simulink model "Swarm"  (Simulink 7.7)
settings: Solver=ode5  StartTime=0.0  StopTime=inf  FixedStep=sample_time  RelTol=1e-3
InitFcn:
  | sample_time=0.005;%0.004;%0.0025;%0.02;
  | sample_time_Vicon = 0.005;
  | DeltaT = 0.02;
  | g = 9.81;
  | H0 = g%0.3165;
  | Kl = 1;
  | 
  | Q6_mass = 0.73;
  | 
  | Q6_Omega_r = 1.5; %for horizon ref
  | Q6_Zeta_r = 0.5; %for horizon ref
  | Q6_Omega_r_h = 2;%for vertical ref
  | Q6_Zeta_r_h = 1; %for vertical ref
  | 
  | Q6_Omega = 1.5; %for horizon control
  | Q6_Zeta = 0.5; %for horizon control
  | Q6_Omega_h= 2; %for vertical control
  | Q6_Zeta_h = 0.7; %for vertical control
  | 
  | Q6_acc_max = 5;%horizontal max acc
  | Q6_acc_max_h = 3;%horizontal max acc
  | 
  | omega_circle = 36*pi/180;
  | omega_h = 0.1;%Ascending speed
  | PI = pi;
  | Circle_R = 2;
  | MAX_Height = -2;
  | 
  | r0=2; %desired separation distance
  | num = 3; %number of neighbors
libraries: X330_Control x22, simulink x16
(part 1 of 2)
settings Model: Creator=ttcl3  LastModifiedBy=Vicon
settings SolverCC: MaxConsecutiveMinStep=auto
settings DebuggingCC: MultiTaskRateTransMsg=warning
settings SFSimCC: SimParseCustomCode=off

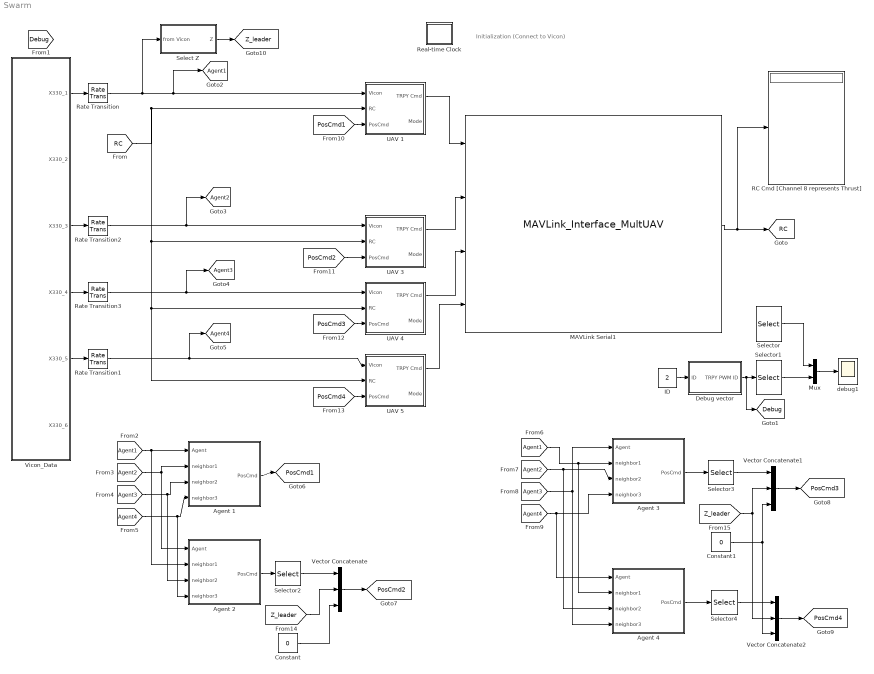
== system Swarm ==
  note: Initialization
      | (Connect to Vicon)
  Agent 1 : Subsystem
  Agent 2 : Subsystem
  Agent 3 : Subsystem
  Agent 4 : Subsystem
  Constant : Constant  Value=0  SampleTime=DeltaT
  Constant1 : Constant  Value=0  SampleTime=DeltaT
  Debug vector : Subsystem
  ID : Constant  Value=2
  MAVLink Serial1 : S-Function  FunctionName=MAVLink_Interface_MultUAV  Parameters=COM_Port,Baud_Rate,MSG_INPUT,MSG_OUTPUT  EnableBusSupport=off  mask{COM_Port='COM7', Baud_Rate=57600, ATTITUDE_OUT=off, RC_SCALED=on, Quad_1=on, Quad_2=off, Quad_3=on, Quad_4=on, Quad_5=on, Quad_6=off, Quad_7=off, Quad_8=off, Quad_9=off, Quad_10=off, Quad_11=off, Quad_12=off, Quad_13=off, Quad_14=off, Quad_15=off, Quad_16=off, Quad_17=off, Quad_18=off, Quad_19=off, Quad_20=off, Quad_21=off, Quad_22=off, Quad_23=off, Quad_24=off, Quad_25=off, Quad_26=off, Quad_27=off, Quad_28=off, Quad_29=off, Quad_30=off}
      mask prompts: COM_Port "COM Port"; Baud_Rate "Baud Rate"; ATTITUDE_OUT "ATTITUDE"; RC_SCALED "RC CHANNELS SCALED"; Quad_1 "Quad No 1"; Quad_2 "Quad No 2"; Quad_3 "Quad No 3"; Quad_4 "Quad No 4"; Quad_5 "Quad No 5"; Quad_6 "Quad No 6"; Quad_7 "Quad No 7"; Quad_8 "Quad No 8"; Quad_9 "Quad No 9"; Quad_10 "Quad No 10"; Quad_11 "Quad No 11"; Quad_12 "Quad No 12"; Quad_13 "Quad No 13"; Quad_14 "Quad No 14"; Quad_15 "Quad No 15"; Quad_16 "Quad No 16"; Quad_17 "Quad No 17"; Quad_18 "Quad No 18"; Quad_19 "Quad No 19"; Quad_20 "Quad No 20"; Quad_21 "Quad No 21"; Quad_22 "Quad No 22"; Quad_23 "Quad No 23"; Quad_24 "Quad No 24"; Quad_25 "Quad No 25"; Quad_26 "Quad No 26"; Quad_27 "Quad No 27"; Quad_28 "Quad No 28"; Quad_29 "Quad No 29"; Quad_30 "Quad No 30"
      mask init:
      | MSG_ID_NUM_INPUT = [uint8(196) uint8(197) uint8(198) uint8(199) uint8(200) uint8(201) uint8(202) uint8(203) uint8(204) uint8(205)
      |                     uint8(206) uint8(207) uint8(208) uint8(209) uint8(210) uint8(211) uint8(212) uint8(213) uint8(214) uint8(215)
      |                     uint8(216) uint8(217) uint8(218) uint8(219) uint8(220) uint8(221) uint8(222) uint8(223) uint8(224) uint8(225)];
      | MSG_ID_NAME_INPUT = [Quad_1 Quad_2 Quad_3 Quad_4 Quad_5 Quad_6 Quad_7 Quad_8 Quad_9 Quad_10
      |                      Quad_11 Quad_12 Quad_13 Quad_14 Quad_15 Quad_16 Quad_17 Quad_18 Quad_19 Quad_20
      |                      Quad_21 Quad_22 Quad_23 Quad_24 Quad_25 Quad_26 Quad_27 Quad_28 Quad_29 Quad_30];
      | 
      | MSG_ID_NUM_OUTPUT = [uint8(34) uint8(30)];
      | MSG_ID_NAME_OUTPUT = [RC_SCALED ATTITUDE_OUT ];
      | 
      | idx_input = find(MSG_ID_NAME_INPUT);
      | MSG_INPUT = MSG_ID_NUM_INPUT(idx_input);
      | 
      | idx_output = find(MSG_ID_NAME_OUTPUT);
      | MSG_OUTPUT = MSG_ID_NUM_OUTPUT(idx_output);
      mask TabNameString: Setting,Setting,Output Message,Output Message,Input Message,Input Message,Input Message,Input Message,Input Message,Input Message,Input Message,Input Message,Input Message,Input Message,Input Message,Input Message,Input Message,Input Message,Input Message,Input Message,Input Message,Input Message,Input Message,Input Message,Input Message,Input Message,Input Message,Input Message,Input Message,Input Message,Input Message,Input Message,Input Message,Input Message
      mask Display:
      | % Block image
      | image(imread('10-inch Quad Heat Map.png'));
      | 
      | %Label block
      | fprintf('MAVLink Serial\n%s\n%dbps', COM_Port,  Baud_Rate)
      | 
      | 
      | %Label input ports
      | 
      | in = 1;
      | if (Quad_1 == 1)
      |     port_label('input', in, 'Quad 1');
      |     in = in + 1;
      | end
      | if (Quad_2 == 1)
      |     port_label('input', in, 'Quad 2');
      |     in = in + 1;
      | end
      | 
      | if (Quad_3 == 1)
      |     port_label('input', in, 'Quad 3');
      |     in = in + 1;
      | end
      | 
      | if (Quad_4 == 1)
      |     port_label('input', in, 'Quad 4');
      |     in = in + 1;
      | end
      | 
      | if (Quad_5 == 1)
      |     port_label('input', in, 'Quad 5');
      |     in = in + 1;
      | end
      | 
      | if (Quad_6 == 1)
      |     port_label('input', in, 'Quad 6');
      |     in = in + 1;
      | end
      | 
      | if (Quad_7 == 1)
      |     port_label('input', in, 'Quad 7');
      |     in = in + 1;
      | end
      | 
      | if (Quad_8 == 1)
      |     port_label('input', in, 'Quad 8');
      |     in = in + 1;
      | end
      | 
      | if (Quad_9 == 1)
      |     port_label('input', in, 'Quad 9');
      |     in = in + 1;
      | end
      | 
      | if (Quad_10 == 1)
      |     port_label('input', in, 'Quad 10');
      |     in = in + 1;
      | end
      | 
      | if (Quad_11 == 1)
      |     port_label('input', in, 'Quad 11');
      |     in = in + 1;
      | end
      | 
      | if (Quad_12 == 1)
      |     port_label('input', in, 'Quad 12');
      |     in = in + 1;
      | end
      | 
      | if (Quad_13 == 1)
      |     port_label('input', in, 'Quad 13');
      |     in = in + 1;
      | end
      | 
      | if (Quad_14 == 1)
      |     port_label('input', in, 'Quad 14');
      |     in = in + 1;
      | end
      | 
      | if (Quad_15 == 1)
      |     port_label('input', in, 'Quad 15');
      |     in = in + 1;
      | end
      | 
      | if (Quad_16 == 1)
      |     port_label('input', in, 'Quad 16');
      |     in = in + 1;
      | end
      | 
      | if (Quad_17 == 1)
      |     port_label('input', in, 'Quad 17');
      |     in = in + 1;
      | end
      | 
      | if (Quad_18 == 1)
      |     port_label('input', in, 'Quad 18');
      |     in = in + 1;
      | end
      | 
      | 
      | if (Quad_19 == 1)
      |     port_label('input', in, 'Quad 19');
      |     in = in + 1;
      | end
      | 
      | if (Quad_20 == 1)
      |     port_label('input', in, 'Quad 20');
      |     in = in + 1;
      | end
      | 
      | if (Quad_21 == 1)
      |     port_label('input', in, 'Quad 21');
      |     in = in + 1;
      | end
      | 
      | if (Quad_22 == 1)
      |     port_label('input', in, 'Quad 22');
      |     in = in + 1;
      | end
      | 
      | if (Quad_23 == 1)
      |     port_label('input', in, 'Quad 23');
      |     in = in + 1;
      | end
      | 
      | if (Quad_24 == 1)
      |     port_label('input', in, 'Quad 24');
      |     in = in + 1;
      | end
      | 
      | if (Quad_25 == 1)
      |     port_label('input', in, 'Quad 25');
      |     in = in + 1;
      | end
      | 
      | if (Quad_26 == 1)
      |     port_label('input', in, 'Quad 26');
      |     in = in + 1;
      | end
      | 
      | if (Quad_27 == 1)
      |     port_label('input', in, 'Quad 27');
      |     in = in + 1;
      | end
      | 
      | if (Quad_28 == 1)
      |     port_label('input', in, 'Quad 28');
      |     in = in + 1;
      | end
      | 
      | if (Quad_29 == 1)
      |     port_label('input', in, 'Quad 29');
      |     in = in + 1;
      | end
      | 
      | if (Quad_30 == 1)
      |     port_label('input', in, 'Quad 30');
      |     in = in + 1;
      | end
      | %Label output ports
      | 
      | out = 1;
      | if (RC_SCALED == 1)
      |     port_label('output', out, 'RC CMD');
      |     out = out + 1;
      | end
      | 
      | if (ATTITUDE_OUT == 1)
      |     port_label('output', out, 'DEBUG');
      |     out = out + 1;
      | end
  Mux : Mux  Inputs=2
  RC Cmd [Channel 8 represents Thrust] : Display
  Rate Transition{,1..3} (4 alike) : RateTransition  OutPortSampleTime=0.02
  Real-time Clock : Subsystem  mask(Real-time Clock){sample_time=0.02, tolerance=1}
      mask prompts: sample_time "Synchronize with real-time every n seconds:"; tolerance "Real-time warning tolerance (seconds):"
      mask help: Real-time Synchronization Block
      mask Help: This block synchronizes simulation time with the PC real-time clock or UNIX system clock. The first dialog entry is the period at which the clock is checked to insure real-time synchronization. The second dialog entry is the number of seconds that the simulation time must be within real-time before a warning is printed.
      mask Display: plot(0,0,100,100,[40,60,60,54,54,64,69,76,82,77,81,83,83,81,78,74,70,64,57,49,41,35,32,30,30,31,34,40,47,47,40,40],[90,90,85,85,80,79,76,87,80,70,64,57,49,41,33,28,24,22,21,23,25,31,37,46,56,65,73,78,80,85,85,90],[69,53,53],[64,50,73])
  Select Z : Subsystem
  Selector : Selector  InputPortWidth=6  IndexOptions=Index vector (dialog)  Indices=[3]  OutputSizes=1
  Selector1 : Selector  InputPortWidth=6  IndexOptions=Index vector (dialog)  Indices=1  OutputSizes=1
  Selector2 : Selector  InputPortWidth=4  IndexOptions=Index vector (dialog)  Indices=[1 2]  OutputSizes=1
  Selector3 : Selector  InputPortWidth=4  IndexOptions=Index vector (dialog)  Indices=[1 2]  OutputSizes=1
  Selector4 : Selector  InputPortWidth=4  IndexOptions=Index vector (dialog)  Indices=[1 2]  OutputSizes=1
  UAV 1 : Subsystem
  UAV 3 : Subsystem
  UAV 4 : Subsystem
  UAV 5 : Subsystem
  Vector Concatenate : Concatenate  NumInputs=3  Mode=Vector
  Vector Concatenate1 : Concatenate  NumInputs=3  Mode=Vector
  Vector Concatenate2 : Concatenate  NumInputs=3  Mode=Vector
  Vicon_Data : Subsystem
  debug1 : Scope
      settings: TimeRange=10  YMin=-1  YMax=1
  tag scope: Agent1=global, Agent2=global, Agent3=global, Agent4=global, Debug=global, PosCmd1=global, PosCmd2=global, PosCmd3=global, PosCmd4=global, RC=global, Z_leader=global
  wires:
  [RC] -> UAV 1/2(RC), UAV 3/2(RC), UAV 4/2(RC), UAV 5/2(RC)
  Vicon_Data/1(X330_1) -> Rate Transition/1
  Rate Transition/1 -> [Agent1], UAV 1/1(Vicon), Select Z/1(from Vicon)
  Rate Transition2/1 -> UAV 3/1(Vicon), [Agent2]
  Rate Transition3/1 -> [Agent3], UAV 4/1(Vicon)
  Vicon_Data/3(X330_3) -> Rate Transition2/1
  Vicon_Data/4(X330_4) -> Rate Transition3/1
  MAVLink Serial1/1 -> RC Cmd [Channel 8 represents Thrust]/1, [RC]
  Mux/1 -> debug1/1
  Debug vector/1(TRPY PWM ID) -> Selector1/1, [Debug]
  ID/1 -> Debug vector/1(ID)
  Selector/1 -> Mux/1
  Selector1/1 -> Mux/2
  UAV 1/1(TRPY Cmd) -> MAVLink Serial1/1
  UAV 3/1(TRPY Cmd) -> MAVLink Serial1/2
  UAV 4/1(TRPY Cmd) -> MAVLink Serial1/3
  Vicon_Data/5(X330_5) -> Rate Transition1/1
  Rate Transition1/1 -> [Agent4], UAV 5/1(Vicon)
  [Agent1] -> Agent 1/1(Agent), Agent 2/2(neighbor1)
  [Agent2] -> Agent 1/2(neighbor1), Agent 2/1(Agent)
  [Agent3] -> Agent 1/3(neighbor2), Agent 2/3(neighbor2)
  [Agent4] -> Agent 1/4(neighbor3), Agent 2/4(neighbor3)
  [Agent3] -> Agent 3/1(Agent), Agent 4/4(neighbor3)
  [Agent1] -> Agent 3/2(neighbor1), Agent 4/2(neighbor1)
  [Agent2] -> Agent 3/3(neighbor2), Agent 4/3(neighbor2)
  [Agent4] -> Agent 3/4(neighbor3), Agent 4/1(Agent)
  Agent 1/1(PosCmd) -> [PosCmd1]
  Agent 2/1(PosCmd) -> Selector2/1
  [PosCmd2] -> UAV 3/3(PosCmd)
  [PosCmd1] -> UAV 1/3(PosCmd)
  [PosCmd3] -> UAV 4/3(PosCmd)
  [PosCmd4] -> UAV 5/3(PosCmd)
  Select Z/1(Z) -> [Z_leader]
  Selector2/1 -> Vector Concatenate/1
  Vector Concatenate/1 -> [PosCmd2]
  [Z_leader] -> Vector Concatenate/2
  Constant/1 -> Vector Concatenate/3
  Selector3/1 -> Vector Concatenate1/1
  Vector Concatenate1/1 -> [PosCmd3]
  [Z_leader] -> Vector Concatenate1/2, Vector Concatenate2/2
  Constant1/1 -> Vector Concatenate1/3, Vector Concatenate2/3
  Agent 3/1(PosCmd) -> Selector3/1
  Selector4/1 -> Vector Concatenate2/1
  Vector Concatenate2/1 -> [PosCmd4]
  Agent 4/1(PosCmd) -> Selector4/1
  UAV 5/1(TRPY Cmd) -> MAVLink Serial1/4

== system Swarm/Agent 1 ==
  Agent : Inport
  neighbor1 : Inport  Port=2
  neighbor2 : Inport  Port=3
  neighbor3 : Inport  Port=4
  Select XYZY : Subsystem
  Select XYZY1 : Subsystem
  Select XYZY2 : Subsystem
  Select XYZY3 : Subsystem
  Swarming : Subsystem
  PosCmd : Outport
  wires:
  Select XYZY/1(XYZY) -> Swarming/1(agent)
  Select XYZY2/1(XYZY) -> Swarming/2(neighbor1)
  Select XYZY1/1(XYZY) -> Swarming/3(neighbor2)
  Agent/1 -> Select XYZY/1(from Vicon)
  Swarming/1(pos_cmd) -> PosCmd/1
  neighbor1/1 -> Select XYZY2/1(from Vicon)
  neighbor2/1 -> Select XYZY1/1(from Vicon)
  neighbor3/1 -> Select XYZY3/1(from Vicon)
  Select XYZY3/1(XYZY) -> Swarming/4(neighbor3)

== system Swarm/Agent 2 ==
  Agent : Inport
  neighbor1 : Inport  Port=2
  neighbor2 : Inport  Port=3
  neighbor3 : Inport  Port=4
  Select XYZY : Subsystem
  Select XYZY1 : Subsystem
  Select XYZY2 : Subsystem
  Select XYZY3 : Subsystem
  Swarming : Subsystem
  PosCmd : Outport
  wires:
  Select XYZY3/1(XYZY) -> Swarming/4(neighbor3)
  neighbor3/1 -> Select XYZY3/1(from Vicon)
  neighbor2/1 -> Select XYZY1/1(from Vicon)
  neighbor1/1 -> Select XYZY2/1(from Vicon)
  Swarming/1(pos_cmd) -> PosCmd/1
  Agent/1 -> Select XYZY/1(from Vicon)
  Select XYZY1/1(XYZY) -> Swarming/3(neighbor2)
  Select XYZY2/1(XYZY) -> Swarming/2(neighbor1)
  Select XYZY/1(XYZY) -> Swarming/1(agent)

== system Swarm/Agent 3 ==
  Agent : Inport
  neighbor1 : Inport  Port=2
  neighbor2 : Inport  Port=3
  neighbor3 : Inport  Port=4
  Select XYZY : Subsystem
  Select XYZY1 : Subsystem
  Select XYZY2 : Subsystem
  Select XYZY3 : Subsystem
  Swarming : Subsystem
  PosCmd : Outport
  wires:
  Select XYZY/1(XYZY) -> Swarming/1(agent)
  Select XYZY2/1(XYZY) -> Swarming/2(neighbor1)
  Select XYZY1/1(XYZY) -> Swarming/3(neighbor2)
  Agent/1 -> Select XYZY/1(from Vicon)
  Swarming/1(pos_cmd) -> PosCmd/1
  neighbor1/1 -> Select XYZY2/1(from Vicon)
  neighbor2/1 -> Select XYZY1/1(from Vicon)
  neighbor3/1 -> Select XYZY3/1(from Vicon)
  Select XYZY3/1(XYZY) -> Swarming/4(neighbor3)

== system Swarm/Agent 4 ==
  Agent : Inport
  neighbor1 : Inport  Port=2
  neighbor2 : Inport  Port=3
  neighbor3 : Inport  Port=4
  Select XYZY : Subsystem
  Select XYZY1 : Subsystem
  Select XYZY2 : Subsystem
  Select XYZY3 : Subsystem
  Swarming : Subsystem
  PosCmd : Outport
  wires:
  Select XYZY3/1(XYZY) -> Swarming/4(neighbor3)
  neighbor3/1 -> Select XYZY3/1(from Vicon)
  neighbor2/1 -> Select XYZY1/1(from Vicon)
  neighbor1/1 -> Select XYZY2/1(from Vicon)
  Swarming/1(pos_cmd) -> PosCmd/1
  Agent/1 -> Select XYZY/1(from Vicon)
  Select XYZY1/1(XYZY) -> Swarming/3(neighbor2)
  Select XYZY2/1(XYZY) -> Swarming/2(neighbor1)
  Select XYZY/1(XYZY) -> Swarming/1(agent)

== system Swarm/Debug vector ==
  note: 6x1 vector (usec, XYZRPY)
  ID : Inport
  Mux1 : Mux  Inputs=6
  PWM : Constant  Value=0
  Pitch : Constant  Value=0
  Roll : Constant  Value=0
  Sine Wave : Sin  SampleTime=0
  Thrust : Constant  Value=0
  Yaw : Constant  Value=0
  TRPY PWM ID : Outport
  wires:
  Mux1/1 -> TRPY PWM ID/1
  Roll/1 -> Mux1/2
  Pitch/1 -> Mux1/3
  Yaw/1 -> Mux1/4
  PWM/1 -> Mux1/5
  ID/1 -> Mux1/6
  Sine Wave/1 -> Mux1/1

== system Swarm/Real-time Clock ==
  Real-time Clock : S-Function  FunctionName=rtclock  Parameters=sample_time, tolerance  EnableBusSupport=off

== system Swarm/Select Z ==
  from Vicon : Inport
  Bus Selector : BusSelector  OutputSignals=Position,Attitude
  Demux : Demux  Outputs=3
  Z : Outport
  wires:
  Bus Selector/1 -> Demux/1  "<Position>"
  from Vicon/1 -> Bus Selector/1
  Demux/3 -> Z/1

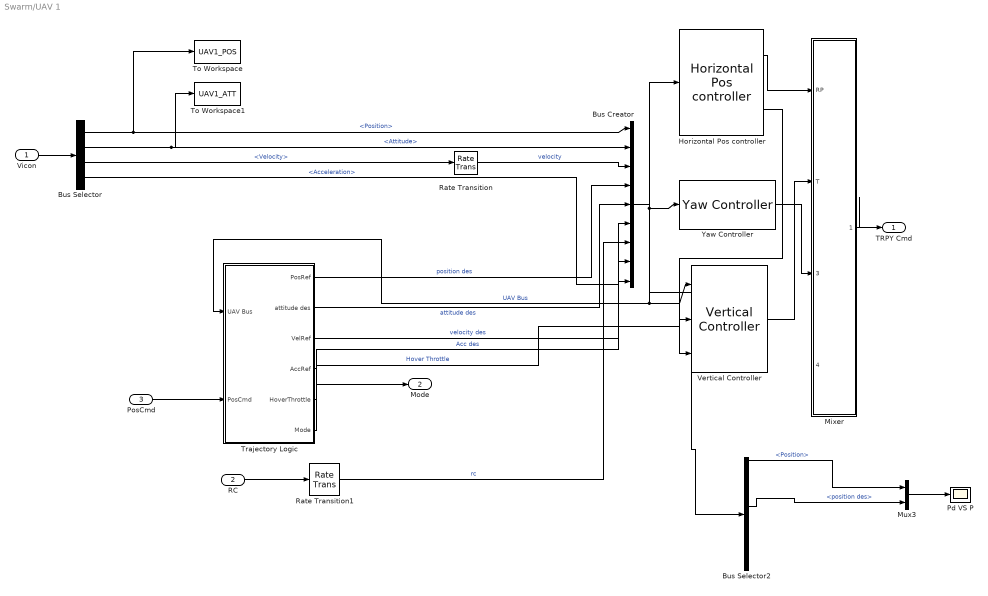
== system Swarm/UAV 1 ==
  Vicon : Inport
  RC : Inport  Port=2
  PosCmd : Inport  Port=3
  Bus Creator : BusCreator  Inputs=9
  Bus Selector : BusSelector  OutputSignals=Position,Attitude,Velocity,Acceleration
  Bus Selector2 : BusSelector  OutputSignals=Position,Attitude,velocity,position des,attitude des,velocity des,rc,Acc des
  Horizontal Pos controller : X330_Control/Horizontal Pos controller  SystemSampleTime=-1  Max_RP=60  Omega=Q6_Omega  PID_i=1  Zeta=Q6_Zeta
  Mixer : Subsystem
  Mux3 : Mux  Inputs=2
  Pd VS P : Scope
      settings: TimeRange=10  YMin=-1.25  YMax=1.75
  Rate Transition : RateTransition  OutPortSampleTime=0.02
  Rate Transition1 : RateTransition  OutPortSampleTime=0.02
  To Workspace : ToWorkspace  VariableName=UAV1_POS  SampleTime=-1  SaveFormat=Structure
  To Workspace1 : ToWorkspace  VariableName=UAV1_ATT  SampleTime=-1  SaveFormat=Structure
  Trajectory Logic : Subsystem
  Vertical Controller : X330_Control/Vertical Controller  SystemSampleTime=-1  Omega_h=Q6_Omega_h  Zeta_h=Q6_Zeta_h  PID_I_h=1  mass=Q6_mass
  Yaw Controller : X330_Control/Yaw Controller  SystemSampleTime=-1
  TRPY Cmd : Outport
  Mode : Outport  Port=2
  wires:
  Mux3/1 -> Pd VS P/1
  Bus Selector2/4 -> Mux3/2  "<position des>"
  Bus Selector2/1 -> Mux3/1  "<Position>"
  Horizontal Pos controller/2 -> Vertical Controller/3
  RC/1 -> Rate Transition1/1
  Trajectory Logic/6(Mode) -> Mode/1
  Trajectory Logic/4(AccRef) -> Bus Creator/9  "Acc des"
  Mixer/1(XYZ RPY) -> TRPY Cmd/1
  Vicon/1 -> Bus Selector/1
  Bus Selector/3 -> Rate Transition/1  "<Velocity>"
  Bus Selector/2 -> Bus Creator/2, To Workspace1/1  "<Attitude>"
  Bus Selector/1 -> To Workspace/1, Bus Creator/1  "<Position>"
  Trajectory Logic/5(HoverThrottle) -> Vertical Controller/2  "Hover Throttle"
  Trajectory Logic/3(VelRef) -> Bus Creator/6  "velocity des"
  Trajectory Logic/2(attitude des) -> Bus Creator/5  "attitude des"
  Trajectory Logic/1(PosRef) -> Bus Creator/4  "position des"
  Bus Selector/4 -> Bus Creator/8  "<Acceleration>"
  Vertical Controller/1 -> Mixer/2(T)
  Yaw Controller/1 -> Mixer/3(Yaw rate)
  Bus Creator/1 -> Yaw Controller/1, Horizontal Pos controller/1, Bus Selector2/1, Vertical Controller/1, Trajectory Logic/1(UAV Bus)  "UAV Bus"
  Rate Transition1/1 -> Bus Creator/7  "rc"
  Rate Transition/1 -> Bus Creator/3  "velocity"
  Horizontal Pos controller/1 -> Mixer/1(RP)
  PosCmd/1 -> Trajectory Logic/2(PosCmd)

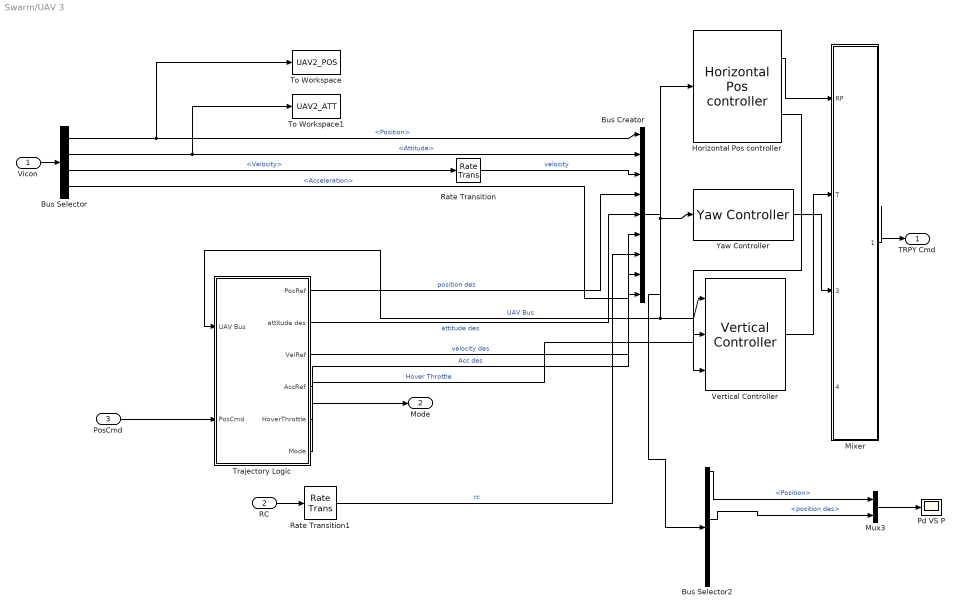
== system Swarm/UAV 3 ==
  Vicon : Inport
  RC : Inport  Port=2
  PosCmd : Inport  Port=3
  Bus Creator : BusCreator  Inputs=9
  Bus Selector : BusSelector  OutputSignals=Position,Attitude,Velocity,Acceleration
  Bus Selector2 : BusSelector  OutputSignals=Position,Attitude,velocity,position des,attitude des,velocity des,rc,Acc des
  Horizontal Pos controller : X330_Control/Horizontal Pos controller  SystemSampleTime=-1  Max_RP=60  Omega=Q6_Omega  PID_i=1  Zeta=Q6_Zeta
  Mixer : Subsystem
  Mux3 : Mux  Inputs=2
  Pd VS P : Scope
      settings: TimeRange=10  YMin=-1.25  YMax=2.75
  Rate Transition : RateTransition  OutPortSampleTime=0.02
  Rate Transition1 : RateTransition  OutPortSampleTime=0.02
  To Workspace : ToWorkspace  VariableName=UAV2_POS  SampleTime=-1  SaveFormat=Structure
  To Workspace1 : ToWorkspace  VariableName=UAV2_ATT  SampleTime=-1  SaveFormat=Structure
  Trajectory Logic : Subsystem
  Vertical Controller : X330_Control/Vertical Controller  SystemSampleTime=-1  Omega_h=Q6_Omega_h  Zeta_h=Q6_Zeta_h  PID_I_h=1  mass=Q6_mass
  Yaw Controller : X330_Control/Yaw Controller  SystemSampleTime=-1
  TRPY Cmd : Outport
  Mode : Outport  Port=2
  wires:
  Mux3/1 -> Pd VS P/1
  Bus Selector2/4 -> Mux3/2  "<position des>"
  Bus Selector2/1 -> Mux3/1  "<Position>"
  Horizontal Pos controller/2 -> Vertical Controller/3
  RC/1 -> Rate Transition1/1
  Trajectory Logic/6(Mode) -> Mode/1
  Trajectory Logic/4(AccRef) -> Bus Creator/9  "Acc des"
  Mixer/1(XYZ RPY) -> TRPY Cmd/1
  Vicon/1 -> Bus Selector/1
  Bus Selector/3 -> Rate Transition/1  "<Velocity>"
  Bus Selector/2 -> Bus Creator/2, To Workspace1/1  "<Attitude>"
  Bus Selector/1 -> Bus Creator/1, To Workspace/1  "<Position>"
  Trajectory Logic/5(HoverThrottle) -> Vertical Controller/2  "Hover Throttle"
  Trajectory Logic/3(VelRef) -> Bus Creator/6  "velocity des"
  Trajectory Logic/2(attitude des) -> Bus Creator/5  "attitude des"
  Trajectory Logic/1(PosRef) -> Bus Creator/4  "position des"
  Bus Selector/4 -> Bus Creator/8  "<Acceleration>"
  Vertical Controller/1 -> Mixer/2(T)
  Yaw Controller/1 -> Mixer/3(Yaw rate)
  Bus Creator/1 -> Yaw Controller/1, Horizontal Pos controller/1, Bus Selector2/1, Vertical Controller/1, Trajectory Logic/1(UAV Bus)  "UAV Bus"
  Rate Transition1/1 -> Bus Creator/7  "rc"
  Rate Transition/1 -> Bus Creator/3  "velocity"
  Horizontal Pos controller/1 -> Mixer/1(RP)
  PosCmd/1 -> Trajectory Logic/2(PosCmd)

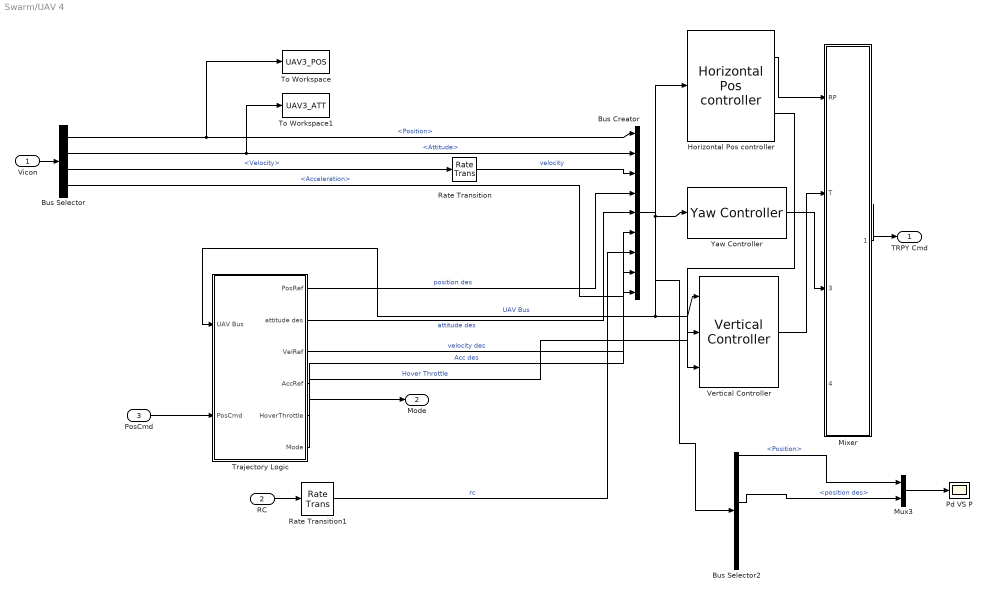
== system Swarm/UAV 4 ==
  Vicon : Inport
  RC : Inport  Port=2
  PosCmd : Inport  Port=3
  Bus Creator : BusCreator  Inputs=9
  Bus Selector : BusSelector  OutputSignals=Position,Attitude,Velocity,Acceleration
  Bus Selector2 : BusSelector  OutputSignals=Position,Attitude,velocity,position des,attitude des,velocity des,rc,Acc des
  Horizontal Pos controller : X330_Control/Horizontal Pos controller  SystemSampleTime=-1  Max_RP=60  Omega=Q6_Omega  PID_i=1  Zeta=Q6_Zeta
  Mixer : Subsystem
  Mux3 : Mux  Inputs=2
  Pd VS P : Scope
      settings: TimeRange=10  YMin=-0.75  YMax=0
  Rate Transition : RateTransition  OutPortSampleTime=0.02
  Rate Transition1 : RateTransition  OutPortSampleTime=0.02
  To Workspace : ToWorkspace  VariableName=UAV3_POS  SampleTime=-1  SaveFormat=Structure
  To Workspace1 : ToWorkspace  VariableName=UAV3_ATT  SampleTime=-1  SaveFormat=Structure
  Trajectory Logic : Subsystem
  Vertical Controller : X330_Control/Vertical Controller  SystemSampleTime=-1  Omega_h=Q6_Omega_h  Zeta_h=Q6_Zeta_h  PID_I_h=1  mass=Q6_mass
  Yaw Controller : X330_Control/Yaw Controller  SystemSampleTime=-1
  TRPY Cmd : Outport
  Mode : Outport  Port=2
  wires:
  Horizontal Pos controller/1 -> Mixer/1(RP)
  Rate Transition/1 -> Bus Creator/3  "velocity"
  Rate Transition1/1 -> Bus Creator/7  "rc"
  Bus Creator/1 -> Trajectory Logic/1(UAV Bus), Vertical Controller/1, Bus Selector2/1, Horizontal Pos controller/1, Yaw Controller/1  "UAV Bus"
  Yaw Controller/1 -> Mixer/3(Yaw rate)
  Vertical Controller/1 -> Mixer/2(T)
  Bus Selector/4 -> Bus Creator/8  "<Acceleration>"
  Trajectory Logic/1(PosRef) -> Bus Creator/4  "position des"
  Trajectory Logic/2(attitude des) -> Bus Creator/5  "attitude des"
  Trajectory Logic/3(VelRef) -> Bus Creator/6  "velocity des"
  Trajectory Logic/5(HoverThrottle) -> Vertical Controller/2  "Hover Throttle"
  Bus Selector/1 -> Bus Creator/1, To Workspace/1  "<Position>"
  Bus Selector/2 -> Bus Creator/2, To Workspace1/1  "<Attitude>"
  Bus Selector/3 -> Rate Transition/1  "<Velocity>"
  Vicon/1 -> Bus Selector/1
  Mixer/1(XYZ RPY) -> TRPY Cmd/1
  Trajectory Logic/4(AccRef) -> Bus Creator/9  "Acc des"
  Trajectory Logic/6(Mode) -> Mode/1
  RC/1 -> Rate Transition1/1
  Horizontal Pos controller/2 -> Vertical Controller/3
  Bus Selector2/1 -> Mux3/1  "<Position>"
  Bus Selector2/4 -> Mux3/2  "<position des>"
  Mux3/1 -> Pd VS P/1
  PosCmd/1 -> Trajectory Logic/2(PosCmd)

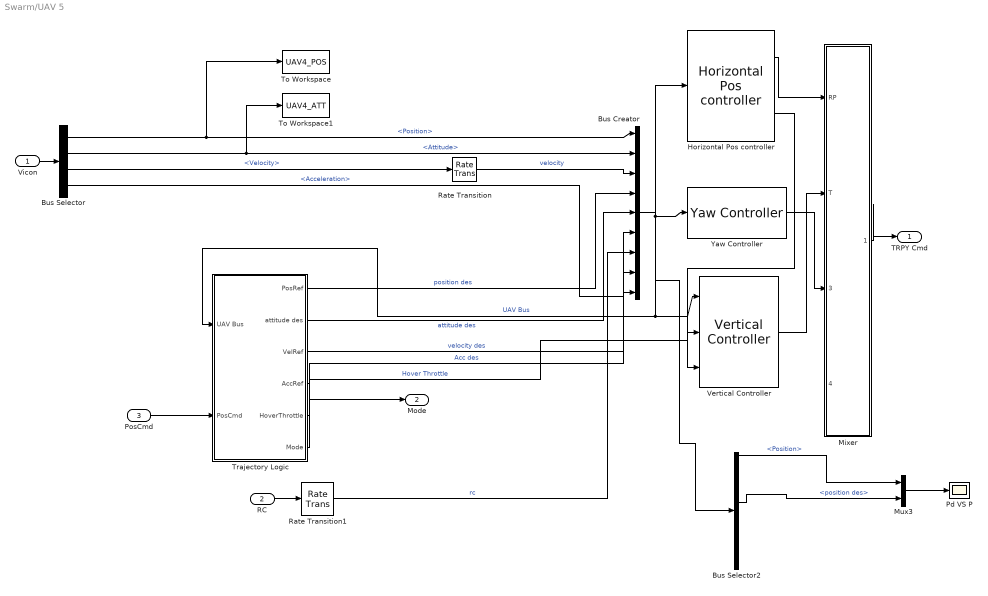
== system Swarm/UAV 5 ==
  Vicon : Inport
  RC : Inport  Port=2
  PosCmd : Inport  Port=3
  Bus Creator : BusCreator  Inputs=9
  Bus Selector : BusSelector  OutputSignals=Position,Attitude,Velocity,Acceleration
  Bus Selector2 : BusSelector  OutputSignals=Position,Attitude,velocity,position des,attitude des,velocity des,rc,Acc des
  Horizontal Pos controller : X330_Control/Horizontal Pos controller  SystemSampleTime=-1  Max_RP=60  Omega=Q6_Omega  PID_i=1  Zeta=Q6_Zeta
  Mixer : Subsystem
  Mux3 : Mux  Inputs=2
  Pd VS P : Scope
      settings: TimeRange=10  YMin=-0.75  YMax=0
  Rate Transition : RateTransition  OutPortSampleTime=0.02
  Rate Transition1 : RateTransition  OutPortSampleTime=0.02
  To Workspace : ToWorkspace  VariableName=UAV4_POS  SampleTime=-1  SaveFormat=Structure
  To Workspace1 : ToWorkspace  VariableName=UAV4_ATT  SampleTime=-1  SaveFormat=Structure
  Trajectory Logic : Subsystem
  Vertical Controller : X330_Control/Vertical Controller  SystemSampleTime=-1  Omega_h=Q6_Omega_h  Zeta_h=Q6_Zeta_h  PID_I_h=1  mass=Q6_mass
  Yaw Controller : X330_Control/Yaw Controller  SystemSampleTime=-1
  TRPY Cmd : Outport
  Mode : Outport  Port=2
  wires:
  PosCmd/1 -> Trajectory Logic/2(PosCmd)
  Mux3/1 -> Pd VS P/1
  Bus Selector2/4 -> Mux3/2  "<position des>"
  Bus Selector2/1 -> Mux3/1  "<Position>"
  Horizontal Pos controller/2 -> Vertical Controller/3
  RC/1 -> Rate Transition1/1
  Trajectory Logic/6(Mode) -> Mode/1
  Trajectory Logic/4(AccRef) -> Bus Creator/9  "Acc des"
  Mixer/1(XYZ RPY) -> TRPY Cmd/1
  Vicon/1 -> Bus Selector/1
  Bus Selector/3 -> Rate Transition/1  "<Velocity>"
  Bus Selector/2 -> To Workspace1/1, Bus Creator/2  "<Attitude>"
  Bus Selector/1 -> To Workspace/1, Bus Creator/1  "<Position>"
  Trajectory Logic/5(HoverThrottle) -> Vertical Controller/2  "Hover Throttle"
  Trajectory Logic/3(VelRef) -> Bus Creator/6  "velocity des"
  Trajectory Logic/2(attitude des) -> Bus Creator/5  "attitude des"
  Trajectory Logic/1(PosRef) -> Bus Creator/4  "position des"
  Bus Selector/4 -> Bus Creator/8  "<Acceleration>"
  Vertical Controller/1 -> Mixer/2(T)
  Yaw Controller/1 -> Mixer/3(Yaw rate)
  Bus Creator/1 -> Yaw Controller/1, Horizontal Pos controller/1, Bus Selector2/1, Vertical Controller/1, Trajectory Logic/1(UAV Bus)  "UAV Bus"
  Rate Transition1/1 -> Bus Creator/7  "rc"
  Rate Transition/1 -> Bus Creator/3  "velocity"
  Horizontal Pos controller/1 -> Mixer/1(RP)

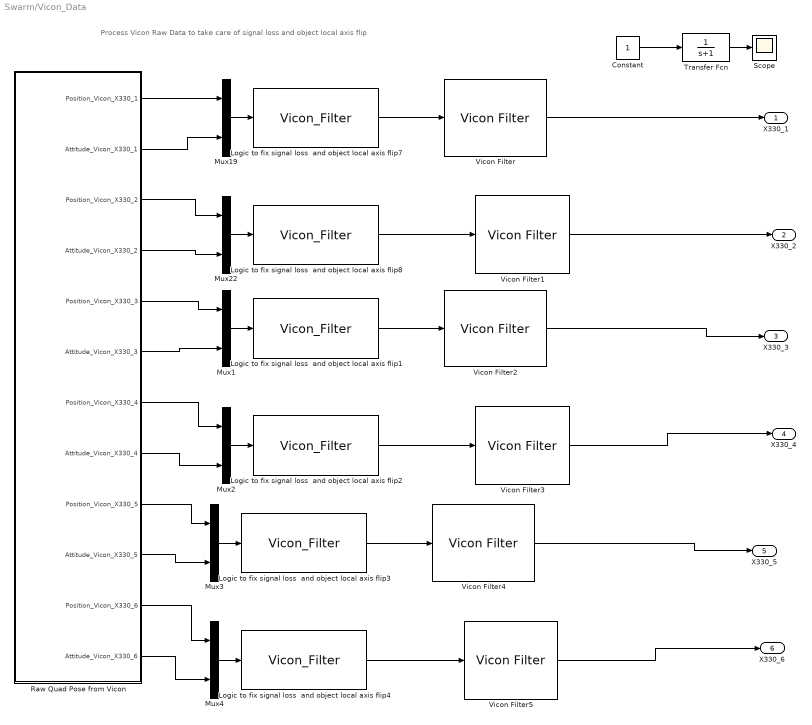
== system Swarm/Vicon_Data ==
  note: Process Vicon Raw Data to take care of signal loss and object local axis flip
  Constant : Constant  SampleTime=5
  Logic to fix signal loss  and object local axis flip{1..4,7..8} (6 alike) : M-S-Function  FunctionName=Vicon_Filter
  Mux{1..4,19,22} (6 alike) : Mux  Inputs=2
  Raw Quad Pose from Vicon : Subsystem
  Scope : Scope
      settings: SaveName=ScopeData2
  Transfer Fcn : TransferFcn  Denominator=[1 1]
  Vicon Filter{,1..5} (6 alike) : X330_Control/Vicon Filter  SystemSampleTime=-1
  X330_1 : Outport
  X330_2 : Outport  Port=2
  X330_3 : Outport  Port=3
  X330_4 : Outport  Port=4
  X330_5 : Outport  Port=5
  X330_6 : Outport  Port=6
  wires:
  Mux19/1 -> Logic to fix signal loss  and object local axis flip7/1
  Mux22/1 -> Logic to fix signal loss  and object local axis flip8/1
  Raw Quad Pose from Vicon/1(Position_Vicon_X330_1) -> Mux19/1
  Raw Quad Pose from Vicon/2(Attitude_Vicon_X330_1) -> Mux19/2
  Raw Quad Pose from Vicon/3(Position_Vicon_X330_2) -> Mux22/1
  Raw Quad Pose from Vicon/4(Attitude_Vicon_X330_2) -> Mux22/2
  Logic to fix signal loss  and object local axis flip7/1 -> Vicon Filter/1
  Vicon Filter/1 -> X330_1/1
  Logic to fix signal loss  and object local axis flip8/1 -> Vicon Filter1/1
  Vicon Filter1/1 -> X330_2/1
  Mux1/1 -> Logic to fix signal loss  and object local axis flip1/1
  Mux2/1 -> Logic to fix signal loss  and object local axis flip2/1
  Logic to fix signal loss  and object local axis flip1/1 -> Vicon Filter2/1
  Vicon Filter2/1 -> X330_3/1
  Logic to fix signal loss  and object local axis flip2/1 -> Vicon Filter3/1
  Vicon Filter3/1 -> X330_4/1
  Mux3/1 -> Logic to fix signal loss  and object local axis flip3/1
  Mux4/1 -> Logic to fix signal loss  and object local axis flip4/1
  Logic to fix signal loss  and object local axis flip3/1 -> Vicon Filter4/1
  Vicon Filter4/1 -> X330_5/1
  Logic to fix signal loss  and object local axis flip4/1 -> Vicon Filter5/1
  Vicon Filter5/1 -> X330_6/1
  Raw Quad Pose from Vicon/5(Position_Vicon_X330_3) -> Mux1/1
  Raw Quad Pose from Vicon/6(Attitude_Vicon_X330_3) -> Mux1/2
  Raw Quad Pose from Vicon/7(Position_Vicon_X330_4) -> Mux2/1
  Raw Quad Pose from Vicon/8(Attitude_Vicon_X330_4) -> Mux2/2
  Raw Quad Pose from Vicon/9(Position_Vicon_X330_5) -> Mux3/1
  Raw Quad Pose from Vicon/10(Attitude_Vicon_X330_5) -> Mux3/2
  Raw Quad Pose from Vicon/11(Position_Vicon_X330_6) -> Mux4/1
  Raw Quad Pose from Vicon/12(Attitude_Vicon_X330_6) -> Mux4/2
  Constant/1 -> Transfer Fcn/1
  Transfer Fcn/1 -> Scope/1

== system Swarm/Agent 1/Select XYZY ==
  from Vicon : Inport
  Bus Selector : BusSelector  OutputSignals=Position,Attitude
  Mux1 : Mux  Inputs=2
  Selector5 : Selector  InputPortWidth=3  IndexOptions=Index vector (dialog)  Indices=[3]  OutputSizes=1
  XYZY : Outport
  wires:
  Selector5/1 -> Mux1/2
  Bus Selector/1 -> Mux1/1  "<Position>"
  Bus Selector/2 -> Selector5/1  "<Attitude>"
  from Vicon/1 -> Bus Selector/1
  Mux1/1 -> XYZY/1

== system Swarm/Agent 1/Select XYZY1 ==
  from Vicon : Inport
  Bus Selector : BusSelector  OutputSignals=Position,Attitude
  Mux1 : Mux  Inputs=2
  Selector5 : Selector  InputPortWidth=3  IndexOptions=Index vector (dialog)  Indices=[3]  OutputSizes=1
  XYZY : Outport
  wires:
  Mux1/1 -> XYZY/1
  from Vicon/1 -> Bus Selector/1
  Bus Selector/2 -> Selector5/1  "<Attitude>"
  Bus Selector/1 -> Mux1/1  "<Position>"
  Selector5/1 -> Mux1/2

== system Swarm/Agent 1/Select XYZY2 ==
  from Vicon : Inport
  Bus Selector : BusSelector  OutputSignals=Position,Attitude
  Mux1 : Mux  Inputs=2
  Selector5 : Selector  InputPortWidth=3  IndexOptions=Index vector (dialog)  Indices=[3]  OutputSizes=1
  XYZY : Outport
  wires:
  Selector5/1 -> Mux1/2
  Bus Selector/1 -> Mux1/1  "<Position>"
  Bus Selector/2 -> Selector5/1  "<Attitude>"
  from Vicon/1 -> Bus Selector/1
  Mux1/1 -> XYZY/1

== system Swarm/Agent 1/Select XYZY3 ==
  from Vicon : Inport
  Bus Selector : BusSelector  OutputSignals=Position,Attitude
  Mux1 : Mux  Inputs=2
  Selector5 : Selector  InputPortWidth=3  IndexOptions=Index vector (dialog)  Indices=[3]  OutputSizes=1
  XYZY : Outport
  wires:
  Selector5/1 -> Mux1/2
  Bus Selector/1 -> Mux1/1  "<Position>"
  Bus Selector/2 -> Selector5/1  "<Attitude>"
  from Vicon/1 -> Bus Selector/1
  Mux1/1 -> XYZY/1

== system Swarm/Agent 1/Swarming ==
  agent : Inport
  neighbor1 : Inport  Port=2
  neighbor2 : Inport  Port=3
  neighbor3 : Inport  Port=4
  Gain2 : Gain  Gain=1/num
  Sum2 : Sum  Inputs=+++
  swarm : Subsystem
  swarm1 : Subsystem
  swarm2 : Subsystem
  pos_cmd : Outport
  wires:
  neighbor2/1 -> swarm1/2(follower)
  agent/1 -> swarm/1(agent), swarm1/1(agent), swarm2/1(agent)
  neighbor1/1 -> swarm/2(follower)
  swarm/1(agent cmd) -> Sum2/1
  swarm1/1(agent cmd) -> Sum2/2
  Sum2/1 -> Gain2/1
  Gain2/1 -> pos_cmd/1
  neighbor3/1 -> swarm2/2(follower)

== system Swarm/Agent 2/Select XYZY ==
  from Vicon : Inport
  Bus Selector : BusSelector  OutputSignals=Position,Attitude
  Mux1 : Mux  Inputs=2
  Selector5 : Selector  InputPortWidth=3  IndexOptions=Index vector (dialog)  Indices=[3]  OutputSizes=1
  XYZY : Outport
  wires:
  Mux1/1 -> XYZY/1
  from Vicon/1 -> Bus Selector/1
  Bus Selector/2 -> Selector5/1  "<Attitude>"
  Bus Selector/1 -> Mux1/1  "<Position>"
  Selector5/1 -> Mux1/2

== system Swarm/Agent 2/Select XYZY1 ==
  from Vicon : Inport
  Bus Selector : BusSelector  OutputSignals=Position,Attitude
  Mux1 : Mux  Inputs=2
  Selector5 : Selector  InputPortWidth=3  IndexOptions=Index vector (dialog)  Indices=[3]  OutputSizes=1
  XYZY : Outport
  wires:
  Selector5/1 -> Mux1/2
  Bus Selector/1 -> Mux1/1  "<Position>"
  Bus Selector/2 -> Selector5/1  "<Attitude>"
  from Vicon/1 -> Bus Selector/1
  Mux1/1 -> XYZY/1

== system Swarm/Agent 2/Select XYZY2 ==
  from Vicon : Inport
  Bus Selector : BusSelector  OutputSignals=Position,Attitude
  Mux1 : Mux  Inputs=2
  Selector5 : Selector  InputPortWidth=3  IndexOptions=Index vector (dialog)  Indices=[3]  OutputSizes=1
  XYZY : Outport
  wires:
  Mux1/1 -> XYZY/1
  from Vicon/1 -> Bus Selector/1
  Bus Selector/2 -> Selector5/1  "<Attitude>"
  Bus Selector/1 -> Mux1/1  "<Position>"
  Selector5/1 -> Mux1/2

== system Swarm/Agent 2/Select XYZY3 ==
  from Vicon : Inport
  Bus Selector : BusSelector  OutputSignals=Position,Attitude
  Mux1 : Mux  Inputs=2
  Selector5 : Selector  InputPortWidth=3  IndexOptions=Index vector (dialog)  Indices=[3]  OutputSizes=1
  XYZY : Outport
  wires:
  Mux1/1 -> XYZY/1
  from Vicon/1 -> Bus Selector/1
  Bus Selector/2 -> Selector5/1  "<Attitude>"
  Bus Selector/1 -> Mux1/1  "<Position>"
  Selector5/1 -> Mux1/2

== system Swarm/Agent 2/Swarming ==
  agent : Inport
  neighbor1 : Inport  Port=2
  neighbor2 : Inport  Port=3
  neighbor3 : Inport  Port=4
  Gain2 : Gain  Gain=1/num
  Sum2 : Sum  Inputs=+++
  swarm : Subsystem
  swarm1 : Subsystem
  swarm2 : Subsystem
  pos_cmd : Outport
  wires:
  neighbor3/1 -> swarm2/2(follower)
  Gain2/1 -> pos_cmd/1
  Sum2/1 -> Gain2/1
  swarm1/1(agent cmd) -> Sum2/2
  swarm/1(agent cmd) -> Sum2/1
  neighbor1/1 -> swarm/2(follower)
  agent/1 -> swarm2/1(agent), swarm1/1(agent), swarm/1(agent)
  neighbor2/1 -> swarm1/2(follower)
  swarm2/1(agent cmd) -> Sum2/3

== system Swarm/Agent 3/Select XYZY ==
  from Vicon : Inport
  Bus Selector : BusSelector  OutputSignals=Position,Attitude
  Mux1 : Mux  Inputs=2
  Selector5 : Selector  InputPortWidth=3  IndexOptions=Index vector (dialog)  Indices=[3]  OutputSizes=1
  XYZY : Outport
  wires:
  Selector5/1 -> Mux1/2
  Bus Selector/1 -> Mux1/1  "<Position>"
  Bus Selector/2 -> Selector5/1  "<Attitude>"
  from Vicon/1 -> Bus Selector/1
  Mux1/1 -> XYZY/1

== system Swarm/Agent 3/Select XYZY1 ==
  from Vicon : Inport
  Bus Selector : BusSelector  OutputSignals=Position,Attitude
  Mux1 : Mux  Inputs=2
  Selector5 : Selector  InputPortWidth=3  IndexOptions=Index vector (dialog)  Indices=[3]  OutputSizes=1
  XYZY : Outport
  wires:
  Mux1/1 -> XYZY/1
  from Vicon/1 -> Bus Selector/1
  Bus Selector/2 -> Selector5/1  "<Attitude>"
  Bus Selector/1 -> Mux1/1  "<Position>"
  Selector5/1 -> Mux1/2

== system Swarm/Agent 3/Select XYZY2 ==
  from Vicon : Inport
  Bus Selector : BusSelector  OutputSignals=Position,Attitude
  Mux1 : Mux  Inputs=2
  Selector5 : Selector  InputPortWidth=3  IndexOptions=Index vector (dialog)  Indices=[3]  OutputSizes=1
  XYZY : Outport
  wires:
  Selector5/1 -> Mux1/2
  Bus Selector/1 -> Mux1/1  "<Position>"
  Bus Selector/2 -> Selector5/1  "<Attitude>"
  from Vicon/1 -> Bus Selector/1
  Mux1/1 -> XYZY/1

== system Swarm/Agent 3/Select XYZY3 ==
  from Vicon : Inport
  Bus Selector : BusSelector  OutputSignals=Position,Attitude
  Mux1 : Mux  Inputs=2
  Selector5 : Selector  InputPortWidth=3  IndexOptions=Index vector (dialog)  Indices=[3]  OutputSizes=1
  XYZY : Outport
  wires:
  Selector5/1 -> Mux1/2
  Bus Selector/1 -> Mux1/1  "<Position>"
  Bus Selector/2 -> Selector5/1  "<Attitude>"
  from Vicon/1 -> Bus Selector/1
  Mux1/1 -> XYZY/1

== system Swarm/Agent 3/Swarming ==
  agent : Inport
  neighbor1 : Inport  Port=2
  neighbor2 : Inport  Port=3
  neighbor3 : Inport  Port=4
  Gain2 : Gain  Gain=1/num
  Sum2 : Sum  Inputs=+++
  swarm : Subsystem
  swarm1 : Subsystem
  swarm2 : Subsystem
  pos_cmd : Outport
  wires:
  neighbor2/1 -> swarm1/2(follower)
  agent/1 -> swarm/1(agent), swarm1/1(agent), swarm2/1(agent)
  neighbor1/1 -> swarm/2(follower)
  swarm/1(agent cmd) -> Sum2/1
  swarm1/1(agent cmd) -> Sum2/2
  Sum2/1 -> Gain2/1
  Gain2/1 -> pos_cmd/1
  neighbor3/1 -> swarm2/2(follower)
  swarm2/1(agent cmd) -> Sum2/3

== system Swarm/Agent 4/Select XYZY ==
  from Vicon : Inport
  Bus Selector : BusSelector  OutputSignals=Position,Attitude
  Mux1 : Mux  Inputs=2
  Selector5 : Selector  InputPortWidth=3  IndexOptions=Index vector (dialog)  Indices=[3]  OutputSizes=1
  XYZY : Outport
  wires:
  Mux1/1 -> XYZY/1
  from Vicon/1 -> Bus Selector/1
  Bus Selector/2 -> Selector5/1  "<Attitude>"
  Bus Selector/1 -> Mux1/1  "<Position>"
  Selector5/1 -> Mux1/2

== system Swarm/Agent 4/Select XYZY1 ==
  from Vicon : Inport
  Bus Selector : BusSelector  OutputSignals=Position,Attitude
  Mux1 : Mux  Inputs=2
  Selector5 : Selector  InputPortWidth=3  IndexOptions=Index vector (dialog)  Indices=[3]  OutputSizes=1
  XYZY : Outport
  wires:
  Selector5/1 -> Mux1/2
  Bus Selector/1 -> Mux1/1  "<Position>"
  Bus Selector/2 -> Selector5/1  "<Attitude>"
  from Vicon/1 -> Bus Selector/1
  Mux1/1 -> XYZY/1

== system Swarm/Agent 4/Select XYZY2 ==
  from Vicon : Inport
  Bus Selector : BusSelector  OutputSignals=Position,Attitude
  Mux1 : Mux  Inputs=2
  Selector5 : Selector  InputPortWidth=3  IndexOptions=Index vector (dialog)  Indices=[3]  OutputSizes=1
  XYZY : Outport
  wires:
  Mux1/1 -> XYZY/1
  from Vicon/1 -> Bus Selector/1
  Bus Selector/2 -> Selector5/1  "<Attitude>"
  Bus Selector/1 -> Mux1/1  "<Position>"
  Selector5/1 -> Mux1/2

== system Swarm/Agent 4/Select XYZY3 ==
  from Vicon : Inport
  Bus Selector : BusSelector  OutputSignals=Position,Attitude
  Mux1 : Mux  Inputs=2
  Selector5 : Selector  InputPortWidth=3  IndexOptions=Index vector (dialog)  Indices=[3]  OutputSizes=1
  XYZY : Outport
  wires:
  Mux1/1 -> XYZY/1
  from Vicon/1 -> Bus Selector/1
  Bus Selector/2 -> Selector5/1  "<Attitude>"
  Bus Selector/1 -> Mux1/1  "<Position>"
  Selector5/1 -> Mux1/2

== system Swarm/Agent 4/Swarming ==
  agent : Inport
  neighbor1 : Inport  Port=2
  neighbor2 : Inport  Port=3
  neighbor3 : Inport  Port=4
  Gain2 : Gain  Gain=1/num
  Sum2 : Sum  Inputs=+++
  swarm : Subsystem
  swarm1 : Subsystem
  swarm2 : Subsystem
  pos_cmd : Outport
  wires:
  neighbor3/1 -> swarm2/2(follower)
  Gain2/1 -> pos_cmd/1
  Sum2/1 -> Gain2/1
  swarm1/1(agent cmd) -> Sum2/2
  swarm/1(agent cmd) -> Sum2/1
  neighbor1/1 -> swarm/2(follower)
  agent/1 -> swarm2/1(agent), swarm1/1(agent), swarm/1(agent)
  neighbor2/1 -> swarm1/2(follower)
  swarm2/1(agent cmd) -> Sum2/3

== system Swarm/UAV 1/Mixer ==
  note: 7x1 vector (usec, XYZRPY)
  RP : Inport
  T : Inport  Port=2
  Yaw rate : Inport  Port=3
  PWM : Inport  Port=4
  Gain : Gain  Gain=180/pi
  Manual Switch : simulink/Signal Routing/Manual Switch  SystemSampleTime=-1  sw=1  action=0  varsize=off
  Mux1 : Mux  Inputs=5
  PWM (1000-close; 2000-open) : Constant  Value=1600  SampleTime=0.02
  PWM (1000-close; 2000-open)1 : Constant  Value=1200  SampleTime=0.02
  "[-1, 1]" : Fcn  Expr=u(1)*2-1
  id : Constant  SampleTime=0.02
  XYZ RPY : Outport
  wires:
  "[-1, 1]"/1 -> Mux1/1
  Gain/1 -> Mux1/2
  PWM/1 -> Mux1/4
  PWM (1000-close; 2000-open)1/1 -> Manual Switch/2
  PWM (1000-close; 2000-open)/1 -> Manual Switch/1
  id/1 -> Mux1/5
  Yaw rate/1 -> Mux1/3
  RP/1 -> Gain/1
  T/1 -> "[-1, 1]"/1
  Mux1/1 -> XYZ RPY/1

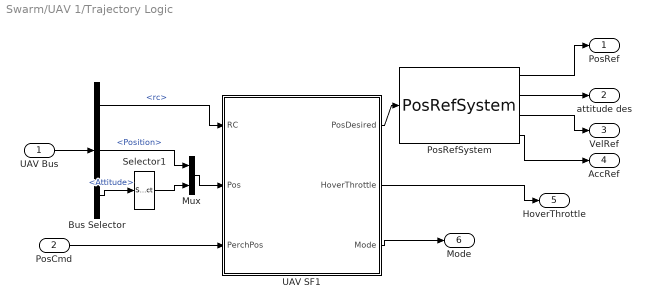
== system Swarm/UAV 1/Trajectory Logic ==
  UAV Bus : Inport
  PosCmd : Inport  Port=2
  Bus Selector : BusSelector  OutputSignals=rc,Position,Attitude
  Mux : Mux  Inputs=2
  PosRefSystem : X330_Control/PosRefSystem  SystemSampleTime=-1  Omega_r=Q6_Omega_r  Zeta_r=Q6_Zeta_r  Acc_Max=Q6_acc_max  Omega_h_r=Q6_Omega_r_h  Zeta_h_r=Q6_Zeta_r_h  Acc_h_Max=Q6_acc_max_h
  Selector1 : Selector  InputPortWidth=3  IndexOptions=Index vector (dialog)  Indices=[3]  OutputSizes=1
  UAV SF1 : Stateflow chart  TreatAsAtomicUnit=on
  PosRef : Outport
  attitude des : Outport  Port=2
  VelRef : Outport  Port=3
  AccRef : Outport  Port=4
  HoverThrottle : Outport  Port=5
  Mode : Outport  Port=6
  wires:
  PosRefSystem/2 -> attitude des/1
  PosRefSystem/4 -> AccRef/1
  PosRefSystem/3 -> VelRef/1
  PosRefSystem/1 -> PosRef/1
  Mux/1 -> UAV SF1/2(Pos)
  Selector1/1 -> Mux/2
  Bus Selector/3 -> Selector1/1  "<Attitude>"
  Bus Selector/2 -> Mux/1  "<Position>"
  UAV Bus/1 -> Bus Selector/1
  UAV SF1/3(Mode) -> Mode/1
  PosCmd/1 -> UAV SF1/3(PerchPos)
  UAV SF1/2(HoverThrottle) -> HoverThrottle/1
  Bus Selector/1 -> UAV SF1/1(RC)  "<rc>"
  UAV SF1/1(PosDesired) -> PosRefSystem/1

== system Swarm/UAV 3/Mixer ==
  note: 7x1 vector (usec, XYZRPY)
  RP : Inport
  T : Inport  Port=2
  Yaw rate : Inport  Port=3
  PWM : Inport  Port=4
  Gain : Gain  Gain=180/pi
  Manual Switch : simulink/Signal Routing/Manual Switch  SystemSampleTime=-1  sw=1  action=0  varsize=off
  Mux1 : Mux  Inputs=5
  PWM (1000-close; 2000-open) : Constant  Value=1600  SampleTime=0.02
  PWM (1000-close; 2000-open)1 : Constant  Value=1200  SampleTime=0.02
  "[-1, 1]" : Fcn  Expr=u(1)*2-1
  id : Constant  Value=3  SampleTime=0.02
  XYZ RPY : Outport
  wires:
  "[-1, 1]"/1 -> Mux1/1
  Gain/1 -> Mux1/2
  PWM/1 -> Mux1/4
  PWM (1000-close; 2000-open)1/1 -> Manual Switch/2
  PWM (1000-close; 2000-open)/1 -> Manual Switch/1
  id/1 -> Mux1/5
  Yaw rate/1 -> Mux1/3
  RP/1 -> Gain/1
  T/1 -> "[-1, 1]"/1
  Mux1/1 -> XYZ RPY/1

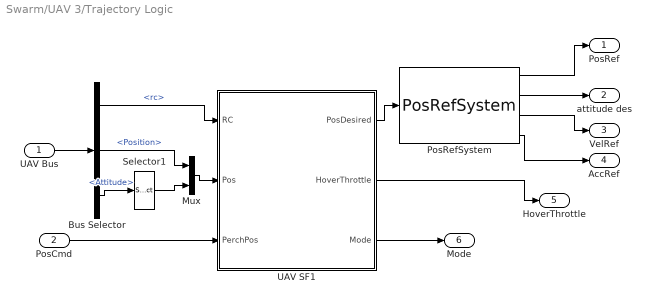
== system Swarm/UAV 3/Trajectory Logic ==
  UAV Bus : Inport
  PosCmd : Inport  Port=2
  Bus Selector : BusSelector  OutputSignals=rc,Position,Attitude
  Mux : Mux  Inputs=2
  PosRefSystem : X330_Control/PosRefSystem  SystemSampleTime=-1  Omega_r=Q6_Omega_r  Zeta_r=Q6_Zeta_r  Acc_Max=Q6_acc_max  Omega_h_r=Q6_Omega_r_h  Zeta_h_r=Q6_Zeta_r_h  Acc_h_Max=Q6_acc_max_h
  Selector1 : Selector  InputPortWidth=3  IndexOptions=Index vector (dialog)  Indices=[3]  OutputSizes=1
  UAV SF1 : Stateflow chart  TreatAsAtomicUnit=on
  PosRef : Outport
  attitude des : Outport  Port=2
  VelRef : Outport  Port=3
  AccRef : Outport  Port=4
  HoverThrottle : Outport  Port=5
  Mode : Outport  Port=6
  wires:
  PosRefSystem/2 -> attitude des/1
  PosRefSystem/4 -> AccRef/1
  PosRefSystem/3 -> VelRef/1
  PosRefSystem/1 -> PosRef/1
  Mux/1 -> UAV SF1/2(Pos)
  Selector1/1 -> Mux/2
  Bus Selector/3 -> Selector1/1  "<Attitude>"
  Bus Selector/2 -> Mux/1  "<Position>"
  UAV Bus/1 -> Bus Selector/1
  UAV SF1/3(Mode) -> Mode/1
  PosCmd/1 -> UAV SF1/3(PerchPos)
  UAV SF1/2(HoverThrottle) -> HoverThrottle/1
  Bus Selector/1 -> UAV SF1/1(RC)  "<rc>"
  UAV SF1/1(PosDesired) -> PosRefSystem/1

== system Swarm/UAV 4/Mixer ==
  note: 7x1 vector (usec, XYZRPY)
  RP : Inport
  T : Inport  Port=2
  Yaw rate : Inport  Port=3
  PWM : Inport  Port=4
  Gain : Gain  Gain=180/pi
  Manual Switch : simulink/Signal Routing/Manual Switch  SystemSampleTime=-1  sw=1  action=0  varsize=off
  Mux1 : Mux  Inputs=5
  PWM (1000-close; 2000-open) : Constant  Value=1600  SampleTime=0.02
  PWM (1000-close; 2000-open)1 : Constant  Value=1200  SampleTime=0.02
  "[-1, 1]" : Fcn  Expr=u(1)*2-1
  id : Constant  Value=4  SampleTime=0.02
  XYZ RPY : Outport
  wires:
  Mux1/1 -> XYZ RPY/1
  T/1 -> "[-1, 1]"/1
  RP/1 -> Gain/1
  Yaw rate/1 -> Mux1/3
  id/1 -> Mux1/5
  PWM (1000-close; 2000-open)/1 -> Manual Switch/1
  PWM (1000-close; 2000-open)1/1 -> Manual Switch/2
  PWM/1 -> Mux1/4
  Gain/1 -> Mux1/2
  "[-1, 1]"/1 -> Mux1/1

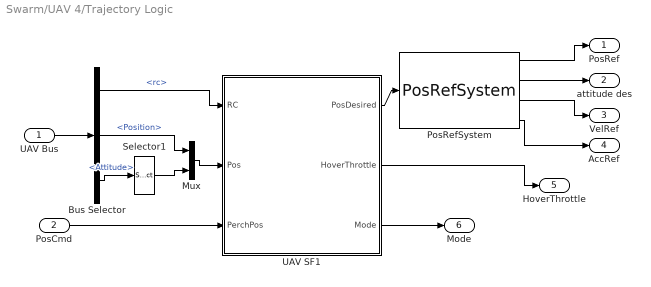
== system Swarm/UAV 4/Trajectory Logic ==
  UAV Bus : Inport
  PosCmd : Inport  Port=2
  Bus Selector : BusSelector  OutputSignals=rc,Position,Attitude
  Mux : Mux  Inputs=2
  PosRefSystem : X330_Control/PosRefSystem  SystemSampleTime=-1  Omega_r=Q6_Omega_r  Zeta_r=Q6_Zeta_r  Acc_Max=Q6_acc_max  Omega_h_r=Q6_Omega_r_h  Zeta_h_r=Q6_Zeta_r_h  Acc_h_Max=Q6_acc_max_h
  Selector1 : Selector  InputPortWidth=3  IndexOptions=Index vector (dialog)  Indices=[3]  OutputSizes=1
  UAV SF1 : Stateflow chart  TreatAsAtomicUnit=on
  PosRef : Outport
  attitude des : Outport  Port=2
  VelRef : Outport  Port=3
  AccRef : Outport  Port=4
  HoverThrottle : Outport  Port=5
  Mode : Outport  Port=6
  wires:
  UAV SF1/1(PosDesired) -> PosRefSystem/1
  Bus Selector/1 -> UAV SF1/1(RC)  "<rc>"
  UAV SF1/2(HoverThrottle) -> HoverThrottle/1
  PosCmd/1 -> UAV SF1/3(PerchPos)
  UAV SF1/3(Mode) -> Mode/1
  UAV Bus/1 -> Bus Selector/1
  Bus Selector/2 -> Mux/1  "<Position>"
  Bus Selector/3 -> Selector1/1  "<Attitude>"
  Selector1/1 -> Mux/2
  Mux/1 -> UAV SF1/2(Pos)
  PosRefSystem/1 -> PosRef/1
  PosRefSystem/3 -> VelRef/1
  PosRefSystem/4 -> AccRef/1
  PosRefSystem/2 -> attitude des/1

== system Swarm/UAV 5/Mixer ==
  note: 7x1 vector (usec, XYZRPY)
  RP : Inport
  T : Inport  Port=2
  Yaw rate : Inport  Port=3
  PWM : Inport  Port=4
  Gain : Gain  Gain=180/pi
  Manual Switch : simulink/Signal Routing/Manual Switch  SystemSampleTime=-1  sw=1  action=0  varsize=off
  Mux1 : Mux  Inputs=5
  PWM (1000-close; 2000-open) : Constant  Value=1600  SampleTime=0.02
  PWM (1000-close; 2000-open)1 : Constant  Value=1200  SampleTime=0.02
  "[-1, 1]" : Fcn  Expr=u(1)*2-1
  id : Constant  Value=5  SampleTime=0.02
  XYZ RPY : Outport
  wires:
  "[-1, 1]"/1 -> Mux1/1
  Gain/1 -> Mux1/2
  PWM/1 -> Mux1/4
  PWM (1000-close; 2000-open)1/1 -> Manual Switch/2
  PWM (1000-close; 2000-open)/1 -> Manual Switch/1
  id/1 -> Mux1/5
  Yaw rate/1 -> Mux1/3
  RP/1 -> Gain/1
  T/1 -> "[-1, 1]"/1
  Mux1/1 -> XYZ RPY/1

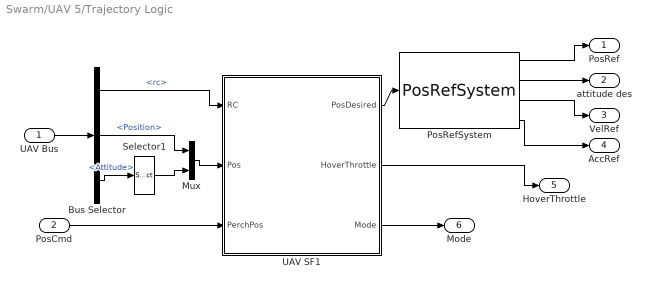
== system Swarm/UAV 5/Trajectory Logic ==
  UAV Bus : Inport
  PosCmd : Inport  Port=2
  Bus Selector : BusSelector  OutputSignals=rc,Position,Attitude
  Mux : Mux  Inputs=2
  PosRefSystem : X330_Control/PosRefSystem  SystemSampleTime=-1  Omega_r=Q6_Omega_r  Zeta_r=Q6_Zeta_r  Acc_Max=Q6_acc_max  Omega_h_r=Q6_Omega_r_h  Zeta_h_r=Q6_Zeta_r_h  Acc_h_Max=Q6_acc_max_h
  Selector1 : Selector  InputPortWidth=3  IndexOptions=Index vector (dialog)  Indices=[3]  OutputSizes=1
  UAV SF1 : Stateflow chart  TreatAsAtomicUnit=on
  PosRef : Outport
  attitude des : Outport  Port=2
  VelRef : Outport  Port=3
  AccRef : Outport  Port=4
  HoverThrottle : Outport  Port=5
  Mode : Outport  Port=6
  wires:
  PosRefSystem/2 -> attitude des/1
  PosRefSystem/4 -> AccRef/1
  PosRefSystem/3 -> VelRef/1
  PosRefSystem/1 -> PosRef/1
  Mux/1 -> UAV SF1/2(Pos)
  Selector1/1 -> Mux/2
  Bus Selector/3 -> Selector1/1  "<Attitude>"
  Bus Selector/2 -> Mux/1  "<Position>"
  UAV Bus/1 -> Bus Selector/1
  UAV SF1/3(Mode) -> Mode/1
  PosCmd/1 -> UAV SF1/3(PerchPos)
  UAV SF1/2(HoverThrottle) -> HoverThrottle/1
  Bus Selector/1 -> UAV SF1/1(RC)  "<rc>"
  UAV SF1/1(PosDesired) -> PosRefSystem/1

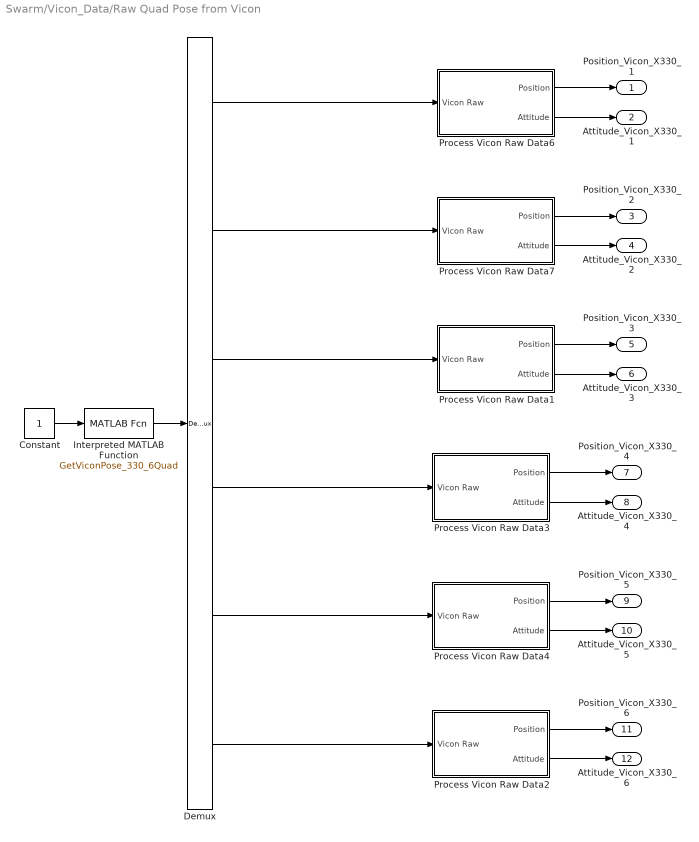
== system Swarm/Vicon_Data/Raw Quad Pose from Vicon ==
  Constant : Constant  SampleTime=sample_time
  Demux : Demux  Outputs=6
  Interpreted MATLAB Function : MATLABFcn  MATLABFcn=GetViconPose_330_6Quad
  Process Vicon Raw Data1 : Subsystem
  Process Vicon Raw Data2 : Subsystem
  Process Vicon Raw Data3 : Subsystem
  Process Vicon Raw Data4 : Subsystem
  Process Vicon Raw Data6 : Subsystem
  Process Vicon Raw Data7 : Subsystem
  Position_Vicon_X330_1 : Outport
  Attitude_Vicon_X330_1 : Outport  Port=2
  Position_Vicon_X330_2 : Outport  Port=3
  Attitude_Vicon_X330_2 : Outport  Port=4
  Position_Vicon_X330_3 : Outport  Port=5
  Attitude_Vicon_X330_3 : Outport  Port=6
  Position_Vicon_X330_4 : Outport  Port=7
  Attitude_Vicon_X330_4 : Outport  Port=8
  Position_Vicon_X330_5 : Outport  Port=9
  Attitude_Vicon_X330_5 : Outport  Port=10
  Position_Vicon_X330_6 : Outport  Port=11
  Attitude_Vicon_X330_6 : Outport  Port=12
  wires:
  Interpreted MATLAB Function/1 -> Demux/1
  Process Vicon Raw Data6/2(Attitude) -> Attitude_Vicon_X330_1/1
  Process Vicon Raw Data6/1(Position) -> Position_Vicon_X330_1/1
  Demux/1 -> Process Vicon Raw Data6/1(Vicon Raw)
  Constant/1 -> Interpreted MATLAB Function/1
  Process Vicon Raw Data7/2(Attitude) -> Attitude_Vicon_X330_2/1
  Process Vicon Raw Data7/1(Position) -> Position_Vicon_X330_2/1
  Demux/2 -> Process Vicon Raw Data7/1(Vicon Raw)
  Process Vicon Raw Data1/2(Attitude) -> Attitude_Vicon_X330_3/1
  Process Vicon Raw Data1/1(Position) -> Position_Vicon_X330_3/1
  Process Vicon Raw Data3/2(Attitude) -> Attitude_Vicon_X330_4/1
  Process Vicon Raw Data3/1(Position) -> Position_Vicon_X330_4/1
  Process Vicon Raw Data4/2(Attitude) -> Attitude_Vicon_X330_5/1
  Process Vicon Raw Data4/1(Position) -> Position_Vicon_X330_5/1
  Process Vicon Raw Data2/2(Attitude) -> Attitude_Vicon_X330_6/1
  Process Vicon Raw Data2/1(Position) -> Position_Vicon_X330_6/1
  Demux/3 -> Process Vicon Raw Data1/1(Vicon Raw)
  Demux/4 -> Process Vicon Raw Data3/1(Vicon Raw)
  Demux/5 -> Process Vicon Raw Data4/1(Vicon Raw)
  Demux/6 -> Process Vicon Raw Data2/1(Vicon Raw)

== system Swarm/Agent 1/Swarming/swarm ==
  agent : Inport
  follower : Inport  Port=2
  2 UAV Swarm Algorithm : Stateflow chart  TreatAsAtomicUnit=on
  Constant : Constant  Value=r0
  agent cmd : Outport
  wires:
  agent/1 -> 2 UAV Swarm Algorithm/1(pos1)
  follower/1 -> 2 UAV Swarm Algorithm/2(pos2)
  2 UAV Swarm Algorithm/2(pos_cmd1) -> agent cmd/1
  Constant/1 -> 2 UAV Swarm Algorithm/3(r0)

== system Swarm/Agent 1/Swarming/swarm1 ==
  agent : Inport
  follower : Inport  Port=2
  2 UAV Swarm Algorithm : Stateflow chart  TreatAsAtomicUnit=on
  Constant : Constant  Value=r0
  agent cmd : Outport
  wires:
  Constant/1 -> 2 UAV Swarm Algorithm/3(r0)
  2 UAV Swarm Algorithm/2(pos_cmd1) -> agent cmd/1
  follower/1 -> 2 UAV Swarm Algorithm/2(pos2)
  agent/1 -> 2 UAV Swarm Algorithm/1(pos1)

== system Swarm/Agent 1/Swarming/swarm2 ==
  agent : Inport
  follower : Inport  Port=2
  2 UAV Swarm Algorithm : Stateflow chart  TreatAsAtomicUnit=on
  Constant : Constant  Value=r0
  agent cmd : Outport
  wires:
  agent/1 -> 2 UAV Swarm Algorithm/1(pos1)
  follower/1 -> 2 UAV Swarm Algorithm/2(pos2)
  2 UAV Swarm Algorithm/2(pos_cmd1) -> agent cmd/1
  Constant/1 -> 2 UAV Swarm Algorithm/3(r0)

== system Swarm/Agent 2/Swarming/swarm ==
  agent : Inport
  follower : Inport  Port=2
  2 UAV Swarm Algorithm : Stateflow chart  TreatAsAtomicUnit=on
  Constant : Constant  Value=r0
  agent cmd : Outport
  wires:
  Constant/1 -> 2 UAV Swarm Algorithm/3(r0)
  2 UAV Swarm Algorithm/2(pos_cmd1) -> agent cmd/1
  follower/1 -> 2 UAV Swarm Algorithm/2(pos2)
  agent/1 -> 2 UAV Swarm Algorithm/1(pos1)

== system Swarm/Agent 2/Swarming/swarm1 ==
  agent : Inport
  follower : Inport  Port=2
  2 UAV Swarm Algorithm : Stateflow chart  TreatAsAtomicUnit=on
  Constant : Constant  Value=r0
  agent cmd : Outport
  wires:
  agent/1 -> 2 UAV Swarm Algorithm/1(pos1)
  follower/1 -> 2 UAV Swarm Algorithm/2(pos2)
  2 UAV Swarm Algorithm/2(pos_cmd1) -> agent cmd/1
  Constant/1 -> 2 UAV Swarm Algorithm/3(r0)
